simulink model "multiRobotWarehouseVFH"  (R2020b)
settings: Solver=VariableStepAuto  StartTime=0.0  StopTime=inf  RelTol=1e-3
values from neighbouring files (symbols this model uses):
  chargingStations = [90,15;90,25;90,37;90,50;90,60]    [example.m]    (also in warehouseInitial.mat = [90  15; 90  25; 90  37; 90  50; 90  60])
  loadingStations = [70,55;58,21;65,5;47,5;40,30]    [example.m]    (also in warehouseInitial.mat = [70  55; 58  21; 65  5; 47  5; 40  30])
  logicalObsMap = logical(getOccupancy(opmap) + mapMatrix)    [createOBS.m]    (also in example.m = createOBS(logicalMap, obstacle, inflation_num); warehouseInitial.mat = [1 1 1 1 1 1 1 1 1 1 1 1 ... (10000 elements, 100x100)])
  numRobots = size(robotPoses, 2)    [VisualizeWarehouseRobots.m]    (also in example.m = size(chargingStations,1); showresult.m; warehouseInitial.mat = 5)
  obstacle = [35,30]    [example.m]    (also in warehouseInitial.mat = [35 30])
  packages = [1,3,4,5,2]    [example.m]    (also in warehouseInitial.mat = [1 3 4 5 2])
  unloadingStations = [20,58;20,72;10,78;30,78;20,92]    [example.m]    (also in warehouseInitial.mat = [20  58; 20  72; 10  78; 30  78; 20  92])
undefined symbols (not defined in the file or in its folder): RobotState
libraries: robotmobilelib x5
settings Model: Creator=fan  LastModifiedBy=fan

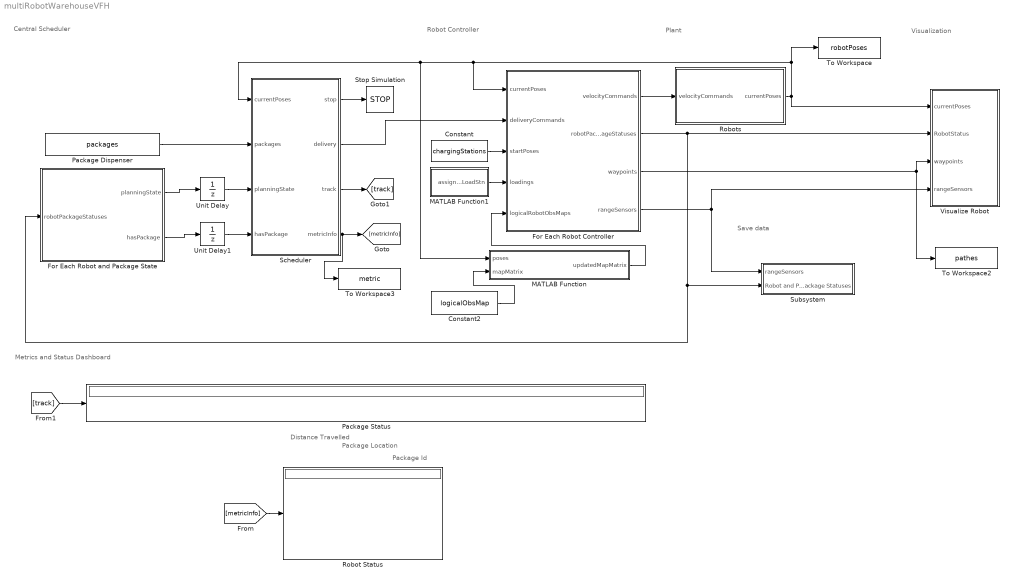
== system multiRobotWarehouseVFH ==
  note: Plant
  note: Package
      | Location
  note: Robot Controller
  note: Metrics and Status Dashboard
  note: Save data
  note: Visualization
  note: Package Id
  note: Distance
      | Travelled
  note: Central Scheduler
  Constant : Constant  Value=chargingStations
  Constant2 : Constant  Value=logicalObsMap
  For Each Robot Controller : Subsystem  TreatAsAtomicUnit=on
  For Each Robot and Package State : Subsystem  TreatAsAtomicUnit=on
  MATLAB Function : MATLAB Function  TreatAsAtomicUnit=on
  MATLAB Function1 : MATLAB Function  TreatAsAtomicUnit=on
  Package Dispenser : Constant  Value=packages
  "Package Status " : Display
  Robot Status : Display
  Robots : Subsystem
  Scheduler : Stateflow chart  Priority=1  TreatAsAtomicUnit=on
  Stop Simulation : Stop
  Subsystem : Subsystem
  To Workspace : ToWorkspace  VariableName=robotPoses  SampleTime=-1
  To Workspace2 : ToWorkspace  VariableName=pathes  SampleTime=-1
  To Workspace3 : ToWorkspace  VariableName=metric  SampleTime=-1
  Unit Delay : UnitDelay  InitialCondition=repmat(RobotState.AtDock, [1, numRobots])  SampleTime=-1  HasFrameUpgradeWarning=on
  Unit Delay1 : UnitDelay  InitialCondition=repmat(0, [1, numRobots])  SampleTime=-1  HasFrameUpgradeWarning=on
  Visualize Robot : Subsystem  mask{MeshSelectionIdx=Ground vehicle, PresetViews=Entire Map, ShowViz=on, ShowPaths=on, MapXMin=0, MapXMax=100, MapYMin=0, MapYMax=100, XLimits=[0 100], YLimits=[0 100], LocalXLimits=[-10 10], LocalYLimits=[-10 10], StartLocations=chargingStations, DockLocations=loadingStations, ShelfLocations=unloadingStations, ObstacleLocation=obstacle, VisualizationSampleRate=10}
      mask prompts: MeshSelectionIdx "Robot mesh"; PresetViews "Preset Views"; ShowViz "Update visualization:"; ShowPaths "Show planned paths:"; MapXMin "Map xmin:"; MapXMax "Map xmax:"; MapYMin "Map ymin:"; MapYMax "Map ymax:"; XLimits "Map x-limits:"; YLimits "Map y-limits:"; LocalXLimits "Local view x-limits"; LocalYLimits "Local view y-limits"; StartLocations "Start locations:"; DockLocations "Dock locations:"; ShelfLocations "Shelf locations:"; ObstacleLocation "Obstacle location:"; VisualizationSampleRate "Sample time:"
      mask init:
      | % Create the list of key locations
      | startLocationMatrix = evalin('base', get_param(gcb, 'StartLocations'));
      | shelfLocationMatrix = evalin('base', get_param(gcb, 'ShelfLocations'));
      | dockLocationMatrix = evalin('base', get_param(gcb, 'DockLocations'));
      | 
      | % Create popup list from matrices
      | dockLocationNameCell = cell(size(dockLocationMatrix,1),1);
      | shelfLocationNameCell = cell(size(shelfLocationMatrix,1),1);
      | startLocationNameCell = cell(size(startLocationMatrix,1),1);
      | for i = 1:size(startLocationMatrix,1)
      |     startLocationNameCell{i} = ['Start Location ' num2str(i)];
      | end
      | for j = 1:size(shelfLocationMatrix,1)
      |     shelfLocationNameCell{j} = ['Shelf Location ' num2str(j)];
      | end
      | for k = 1:size(dockLocationMatrix,1)
      |     dockLocationNameCell{k} = ['Dock Location ' num2str(k)];
      | end
      | 
      | % Update the parameter list
      | m = Simulink.Mask.get(gcb);
      | viewPopupParam = m.getParameter('PresetViews');
      | viewPopupParam.TypeOptions = [...
      |     {'Entire Map'}; ...
      |     dockLocationNameCell; ...
      |     shelfLocationNameCell; ...
      |     startLocationNameCell ... 
      |     ];
      mask TypeOptions MeshSelectionIdx: Ground vehicle | Forklift
      mask TypeOptions PresetViews: Entire Map | Dock Location 1 | Dock Location 2 | Dock Location 3 | Dock Location 4 | Dock Location 5 | Shelf Location 1 | Shelf Location 2 | Shelf Location 3 | Shelf Location 4 | Shelf Location 5 | Start Location 1 | Start Location 2 | Start Location 3 | Start Location 4 | Start Location 5
      mask Callback PresetViews:
      | % Get key numeric data
      | startLocationMatrix = evalin('base', get_param(gcb, 'StartLocations'));
      | dockLocationMatrix = evalin('base', get_param(gcb, 'DockLocations'));
      | shelfLocationMatrix = evalin('base', get_param(gcb, 'ShelfLocations'));
      | mapXLim = evalin('base', get_param(gcb, 'XLimits'));
      | mapYLim = evalin('base', get_param(gcb, 'YLimits'));
      | viewXLim = evalin('base', get_param(gcb, 'LocalXLimits'));
      | viewYLim = evalin('base', get_param(gcb, 'LocalYLimits'));
      | 
      | % Get selected value
      | viewSelection = get_param(gcb, 'PresetViews');
      | 
      | % Take action based on view
      | if strcmp(viewSelection, 'Custom')
      |     % Do nothing
      | else
      |     if strcmp(viewSelection(1:5), 'Start')
      |         % Start location
      |         startIndex = str2double(viewSelection(16:end));
      |         localPts = startLocationMatrix(startIndex, :);
      |         viewLimits = [localPts(1)+viewXLim(1) localPts(1)+viewXLim(2) ...
      |             localPts(2)+viewYLim(1) localPts(2)+viewYLim(2)];
      | 
      |     elseif strcmp(viewSelection(1:5), 'Dock ')
      |         % Dock (Loading) location
      |         dockIndex = str2double(viewSelection(15:end));
      |         localPts = dockLocationMatrix(dockIndex, :);
      |         viewLimits = [localPts(1)+viewXLim(1) localPts(1)+viewXLim(2) ...
      |             localPts(2)+viewYLim(1) localPts(2)+viewYLim(2)];
      | 
      |     elseif strcmp(viewSelection(1:5), 'Shelf')
      |         % Shelf (Unloading) location
      |         shelfIndex = str2double(viewSelection(16:end));
      |         localPts = shelfLocationMatrix(shelfIndex, :);
      |         viewLimits = [localPts(1)+viewXLim(1) localPts(1)+viewXLim(2) ...
      |             localPts(2)+viewYLim(1) localPts(2)+viewYLim(2)];
      | 
      |     else
      |         % Show the whole map
      |         viewLimits = [mapXLim(1) mapXLim(2) mapYLim(1) mapYLim(2)];
      |     end
      | 
      |     % Set the map parameters
      |     set_param(gcb, 'MapXMin', num2str(viewLimits(1)));
      |     set_param(gcb, 'MapXMax', num2str(viewLimits(2)));
      |     set_param(gcb, 'MapYMin', num2str(viewLimits(3)));
      |     set_param(gcb, 'MapYMax', num2str(viewLimits(4)));
      | end
      mask Callback MapXMin:
      | currentMax = str2num(get_param(gcb, 'MapXMax'));
      | newMin = str2num(get_param(gcb, 'MapXMin'));
      | if newMin > currentMax
      |     set_param(gcb, 'MapXMax', num2str(newMin+1));
      | end
      mask Callback MapXMax:
      | currentMin = str2num(get_param(gcb, 'MapXMin'));
      | newMax = str2num(get_param(gcb, 'MapXMax'));
      | if newMax < currentMin
      |     set_param(gcb, 'MapXMin', num2str(newMax-1));
      | end
      mask Callback MapYMin:
      | currentMax = str2num(get_param(gcb, 'MapYMax'));
      | newMin = str2num(get_param(gcb, 'MapYMin'));
      | if newMin > currentMax
      |     set_param(gcb, 'MapYMax', num2str(newMin+1));
      | end
      mask Callback MapYMax:
      | currentMin = str2num(get_param(gcb, 'MapYMin'));
      | newMax = str2num(get_param(gcb, 'MapYMax'));
      | if newMax < currentMin
      |     set_param(gcb, 'MapYMin', num2str(newMax-1));
      | end
      mask DialogControl DescGroupVar Prompt: Visualization example helper
      mask DialogControl DescTextVar Prompt: This subsystem plots the robots and environement and allows users to change the views.
      mask DialogControl ViewLimits Prompt: View limits
      mask DialogControl ViewConfigurationGroup Prompt: View configuration:
      mask DialogControl ViewParamSourcesGroup Prompt: View parameter sources
      mask Display: disp('Visualization Helper')
  wires:
  For Each Robot Controller/4(rangeSensors) -> Subsystem/1(rangeSensors), Visualize Robot/4(rangeSensors)
  Constant2/1 -> MATLAB Function/2(mapMatrix)
  For Each Robot Controller/1(velocityCommands) -> Robots/1(velocityCommands)
  Scheduler/2(delivery) -> For Each Robot Controller/2(deliveryCommands)
  MATLAB Function1/1(assignedLoadStn) -> For Each Robot Controller/4(loadings)
  Unit Delay/1 -> Scheduler/3(planningState)
  For Each Robot and Package State/2(hasPackage) -> Unit Delay1/1
  Unit Delay1/1 -> Scheduler/4(hasPackage)
  [track] -> "Package Status "/1
  Package Dispenser/1 -> Scheduler/2(packages)
  For Each Robot and Package State/1(planningState) -> Unit Delay/1
  Scheduler/1(stop) -> Stop Simulation/1
  For Each Robot Controller/2(robotPackageStatuses) -> Visualize Robot/2(RobotStatus), For Each Robot and Package State/1(robotPackageStatuses), Subsystem/2(Robot and Package Statuses)
  Scheduler/4(metricInfo) -> To Workspace3/1, [metricInfo]
  Constant/1 -> For Each Robot Controller/3(startPoses)
  For Each Robot Controller/3(waypoints) -> To Workspace2/1, Visualize Robot/3(waypoints)
  MATLAB Function/1(updatedMapMatrix) -> For Each Robot Controller/5(logicalRobotObsMaps)
  Robots/1(currentPoses) -> Visualize Robot/1(currentPoses), To Workspace/1, MATLAB Function/1(poses), Scheduler/1(currentPoses), For Each Robot Controller/1(currentPoses)
  [metricInfo] -> Robot Status/1
  Scheduler/3(track) -> [track]

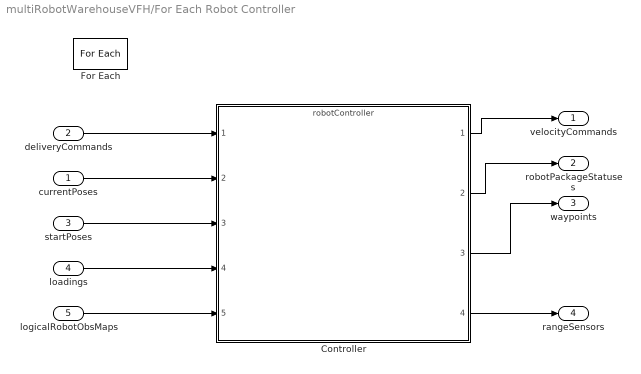
== system multiRobotWarehouseVFH/For Each Robot Controller ==
  currentPoses : Inport  Partition=on  PartitionDimension=2  PartitionWidth=1  PartitionOffset=0
  deliveryCommands : Inport  Port=2  Partition=on  PartitionDimension=1  PartitionWidth=1  PartitionOffset=0
  startPoses : Inport  Port=3  Partition=on  PartitionDimension=1  PartitionWidth=1  PartitionOffset=0
  loadings : Inport  Port=4  Partition=on  PartitionDimension=1  PartitionWidth=1  PartitionOffset=0
  logicalRobotObsMaps : Inport  Port=5  OutDataTypeStr=boolean
  Controller : ModelReference  ModelNameDialog=robotController.slx  ModelReferenceVersion=1.160
  For Each : ForEach  DisableCoverage=on
  velocityCommands : Outport  ConcatenationDimension=2
  robotPackageStatuses : Outport  Port=2  ConcatenationDimension=1
  waypoints : Outport  Port=3  ConcatenationDimension=3
  rangeSensors : Outport  Port=4  ConcatenationDimension=1
  wires:
  deliveryCommands/1 -> Controller/1
  currentPoses/1 -> Controller/2
  startPoses/1 -> Controller/3
  Controller/1 -> velocityCommands/1
  Controller/2 -> robotPackageStatuses/1
  Controller/3 -> waypoints/1
  loadings/1 -> Controller/4
  logicalRobotObsMaps/1 -> Controller/5
  Controller/4 -> rangeSensors/1

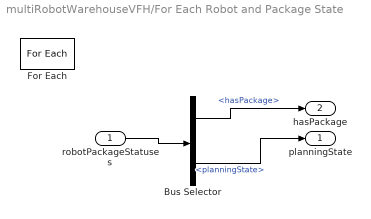
== system multiRobotWarehouseVFH/For Each Robot and Package State ==
  robotPackageStatuses : Inport  Partition=on  PartitionDimension=1  PartitionWidth=1  PartitionOffset=0
  Bus Selector : BusSelector  OutputSignals=hasPackage,planningState
  For Each : ForEach  DisableCoverage=on
  planningState : Outport  ConcatenationDimension=1
  hasPackage : Outport  Port=2  ConcatenationDimension=1
  wires:
  robotPackageStatuses/1 -> Bus Selector/1
  Bus Selector/1 -> hasPackage/1  "<hasPackage>"
  Bus Selector/2 -> planningState/1  "<planningState>"

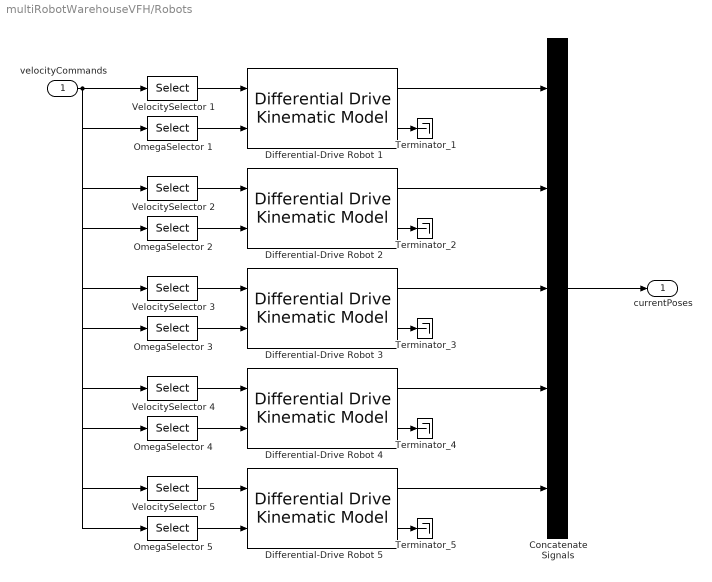
== system multiRobotWarehouseVFH/Robots ==
  velocityCommands : Inport
  Concatenate Signals : Concatenate  NumInputs=5  Mode=Multidimensional array  ConcatenateDimension=2
  Differential-Drive Robot 1 : robotmobilelib/Differential Drive Kinematic Model  VehicleInputs=Vehicle Speed & Heading Angular Velocity  WheelRadius=0.1  WheelSpeedRange=[-inf inf]  TrackWidth=0.2  InitialState=[chargingStations(1, :), 0]'  SimulateUsing=Interpreted execution
      settings: SourceProductName=Robotics System Toolbox
  Differential-Drive Robot 2 : robotmobilelib/Differential Drive Kinematic Model  VehicleInputs=Vehicle Speed & Heading Angular Velocity  WheelRadius=0.1  WheelSpeedRange=[-inf inf]  TrackWidth=0.2  InitialState=[chargingStations(2, :), 0]'  SimulateUsing=Interpreted execution
      settings: SourceProductName=Robotics System Toolbox
  Differential-Drive Robot 3 : robotmobilelib/Differential Drive Kinematic Model  VehicleInputs=Vehicle Speed & Heading Angular Velocity  WheelRadius=0.1  WheelSpeedRange=[-inf inf]  TrackWidth=0.2  InitialState=[chargingStations(3, :), 0]'  SimulateUsing=Interpreted execution
      settings: SourceProductName=Robotics System Toolbox
  Differential-Drive Robot 4 : robotmobilelib/Differential Drive Kinematic Model  VehicleInputs=Vehicle Speed & Heading Angular Velocity  WheelRadius=0.1  WheelSpeedRange=[-inf inf]  TrackWidth=0.2  InitialState=[chargingStations(4, :), 0]'  SimulateUsing=Interpreted execution
      settings: SourceProductName=Robotics System Toolbox
  Differential-Drive Robot 5 : robotmobilelib/Differential Drive Kinematic Model  VehicleInputs=Vehicle Speed & Heading Angular Velocity  WheelRadius=0.1  WheelSpeedRange=[-inf inf]  TrackWidth=0.2  InitialState=[chargingStations(5, :), 0]'  SimulateUsing=Interpreted execution
      settings: SourceProductName=Robotics System Toolbox
  OmegaSelector 1 : Selector  NumberOfDimensions=2  InputPortWidth=3  IndexOptions=Index vector (dialog),Index vector (dialog)  Indices=2,1  OutputSizes=1
  OmegaSelector 2 : Selector  NumberOfDimensions=2  InputPortWidth=3  IndexOptions=Index vector (dialog),Index vector (dialog)  Indices=2,2  OutputSizes=1
  OmegaSelector 3 : Selector  NumberOfDimensions=2  InputPortWidth=3  IndexOptions=Index vector (dialog),Index vector (dialog)  Indices=2,3  OutputSizes=1
  OmegaSelector 4 : Selector  NumberOfDimensions=2  InputPortWidth=3  IndexOptions=Index vector (dialog),Index vector (dialog)  Indices=2,4  OutputSizes=1
  OmegaSelector 5 : Selector  NumberOfDimensions=2  InputPortWidth=3  IndexOptions=Index vector (dialog),Index vector (dialog)  Indices=2,5  OutputSizes=1
  Terminator_{1..5} (5 alike) : Terminator
  VelocitySelector 1 : Selector  NumberOfDimensions=2  InputPortWidth=3  IndexOptions=Index vector (dialog),Index vector (dialog)  Indices=1,1  OutputSizes=1
  VelocitySelector 2 : Selector  NumberOfDimensions=2  InputPortWidth=3  IndexOptions=Index vector (dialog),Index vector (dialog)  Indices=1,2  OutputSizes=1
  VelocitySelector 3 : Selector  NumberOfDimensions=2  InputPortWidth=3  IndexOptions=Index vector (dialog),Index vector (dialog)  Indices=1,3  OutputSizes=1
  VelocitySelector 4 : Selector  NumberOfDimensions=2  InputPortWidth=3  IndexOptions=Index vector (dialog),Index vector (dialog)  Indices=1,4  OutputSizes=1
  VelocitySelector 5 : Selector  NumberOfDimensions=2  InputPortWidth=3  IndexOptions=Index vector (dialog),Index vector (dialog)  Indices=1,5  OutputSizes=1
  currentPoses : Outport
  wires:
  Concatenate Signals/1 -> currentPoses/1
  velocityCommands/1 -> VelocitySelector 1/1, OmegaSelector 1/1, VelocitySelector 2/1, OmegaSelector 2/1, VelocitySelector 3/1, OmegaSelector 3/1, VelocitySelector 4/1, OmegaSelector 4/1, VelocitySelector 5/1, OmegaSelector 5/1
  VelocitySelector 1/1 -> Differential-Drive Robot 1/1
  OmegaSelector 1/1 -> Differential-Drive Robot 1/2
  Differential-Drive Robot 1/1 -> Concatenate Signals/1
  VelocitySelector 2/1 -> Differential-Drive Robot 2/1
  OmegaSelector 2/1 -> Differential-Drive Robot 2/2
  Differential-Drive Robot 2/1 -> Concatenate Signals/2
  VelocitySelector 3/1 -> Differential-Drive Robot 3/1
  OmegaSelector 3/1 -> Differential-Drive Robot 3/2
  Differential-Drive Robot 3/1 -> Concatenate Signals/3
  VelocitySelector 4/1 -> Differential-Drive Robot 4/1
  OmegaSelector 4/1 -> Differential-Drive Robot 4/2
  Differential-Drive Robot 4/1 -> Concatenate Signals/4
  VelocitySelector 5/1 -> Differential-Drive Robot 5/1
  OmegaSelector 5/1 -> Differential-Drive Robot 5/2
  Differential-Drive Robot 5/1 -> Concatenate Signals/5
  Differential-Drive Robot 1/2 -> Terminator_1/1
  Differential-Drive Robot 2/2 -> Terminator_2/1
  Differential-Drive Robot 3/2 -> Terminator_3/1
  Differential-Drive Robot 4/2 -> Terminator_4/1
  Differential-Drive Robot 5/2 -> Terminator_5/1

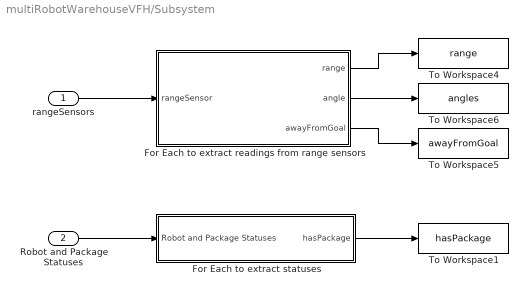
== system multiRobotWarehouseVFH/Subsystem ==
  rangeSensors : Inport
  Robot and Package Statuses : Inport  Port=2
  For Each to extract readings from range sensors : Subsystem  TreatAsAtomicUnit=on
  For Each to extract statuses : Subsystem  TreatAsAtomicUnit=on
  To Workspace1 : ToWorkspace  VariableName=hasPackage  SampleTime=-1
  To Workspace4 : ToWorkspace  VariableName=range  SampleTime=-1
  To Workspace5 : ToWorkspace  VariableName=awayFromGoal  SampleTime=-1
  To Workspace6 : ToWorkspace  VariableName=angles  SampleTime=-1
  wires:
  For Each to extract readings from range sensors/2(angle) -> To Workspace6/1
  For Each to extract readings from range sensors/3(awayFromGoal) -> To Workspace5/1
  For Each to extract readings from range sensors/1(range) -> To Workspace4/1
  rangeSensors/1 -> For Each to extract readings from range sensors/1(rangeSensor)
  For Each to extract statuses/1(hasPackage) -> To Workspace1/1
  Robot and Package Statuses/1 -> For Each to extract statuses/1(Robot and Package Statuses)

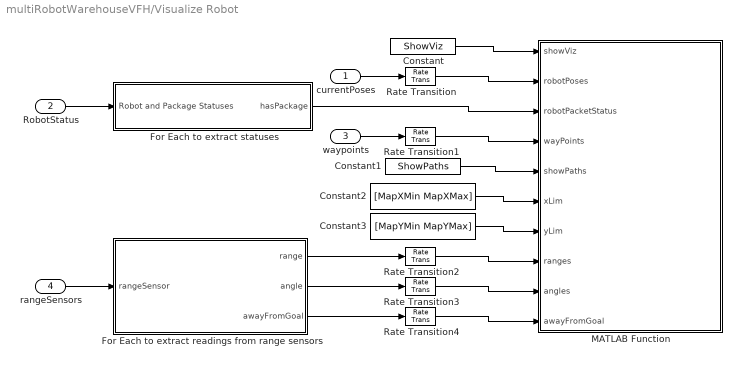
== system multiRobotWarehouseVFH/Visualize Robot ==
  currentPoses : Inport
  RobotStatus : Inport  Port=2
  waypoints : Inport  Port=3
  rangeSensors : Inport  Port=4
  Constant : Constant  Value=ShowViz
  Constant1 : Constant  Value=ShowPaths
  Constant2 : Constant  Value=[MapXMin MapXMax]
  Constant3 : Constant  Value=[MapYMin MapYMax]
  For Each to extract readings from range sensors : Subsystem  TreatAsAtomicUnit=on
  For Each to extract statuses : Subsystem  TreatAsAtomicUnit=on
  MATLAB Function : MATLAB Function  TreatAsAtomicUnit=on
  Rate Transition{,1..4} (5 alike) : RateTransition
  wires:
  waypoints/1 -> Rate Transition1/1
  currentPoses/1 -> Rate Transition/1
  Rate Transition/1 -> MATLAB Function/2(robotPoses)
  Rate Transition1/1 -> MATLAB Function/4(wayPoints)
  Constant/1 -> MATLAB Function/1(showViz)
  Constant1/1 -> MATLAB Function/5(showPaths)
  Constant2/1 -> MATLAB Function/6(xLim)
  Constant3/1 -> MATLAB Function/7(yLim)
  RobotStatus/1 -> For Each to extract statuses/1(Robot and Package Statuses)
  For Each to extract statuses/1(hasPackage) -> MATLAB Function/3(robotPacketStatus)
  For Each to extract readings from range sensors/1(range) -> Rate Transition2/1
  Rate Transition2/1 -> MATLAB Function/8(ranges)
  Rate Transition3/1 -> MATLAB Function/9(angles)
  For Each to extract readings from range sensors/2(angle) -> Rate Transition3/1
  Rate Transition4/1 -> MATLAB Function/10(awayFromGoal)
  For Each to extract readings from range sensors/3(awayFromGoal) -> Rate Transition4/1
  rangeSensors/1 -> For Each to extract readings from range sensors/1(rangeSensor)

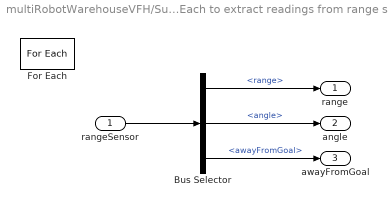
== system multiRobotWarehouseVFH/Subsystem/For Each to extract readings from range sensors ==
  rangeSensor : Inport  Partition=on  PartitionDimension=1  PartitionWidth=1  PartitionOffset=0
  Bus Selector : BusSelector  OutputSignals=range,angle,awayFromGoal
  For Each : ForEach  DisableCoverage=on
  range : Outport  ConcatenationDimension=2
  angle : Outport  Port=2  ConcatenationDimension=2
  awayFromGoal : Outport  Port=3  OutDataTypeStr=boolean  ConcatenationDimension=1
  wires:
  rangeSensor/1 -> Bus Selector/1
  Bus Selector/1 -> range/1  "<range>"
  Bus Selector/2 -> angle/1  "<angle>"
  Bus Selector/3 -> awayFromGoal/1  "<awayFromGoal>"

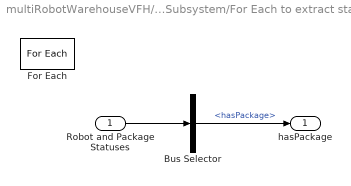
== system multiRobotWarehouseVFH/Subsystem/For Each to extract statuses ==
  Robot and Package Statuses : Inport  Partition=on  PartitionDimension=1  PartitionWidth=1  PartitionOffset=0
  Bus Selector : BusSelector  OutputSignals=hasPackage
  For Each : ForEach  DisableCoverage=on
  hasPackage : Outport  ConcatenationDimension=1
  wires:
  Robot and Package Statuses/1 -> Bus Selector/1
  Bus Selector/1 -> hasPackage/1  "<hasPackage>"

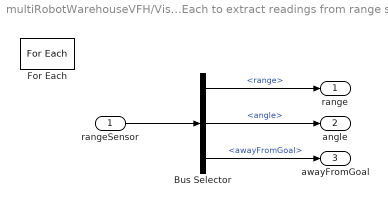
== system multiRobotWarehouseVFH/Visualize Robot/For Each to extract readings from range sensors ==
  rangeSensor : Inport  Partition=on  PartitionDimension=1  PartitionWidth=1  PartitionOffset=0
  Bus Selector : BusSelector  OutputSignals=range,angle,awayFromGoal
  For Each : ForEach  DisableCoverage=on
  range : Outport  ConcatenationDimension=2
  angle : Outport  Port=2  ConcatenationDimension=2
  awayFromGoal : Outport  Port=3  OutDataTypeStr=boolean  ConcatenationDimension=1
  wires:
  rangeSensor/1 -> Bus Selector/1
  Bus Selector/1 -> range/1  "<range>"
  Bus Selector/2 -> angle/1  "<angle>"
  Bus Selector/3 -> awayFromGoal/1  "<awayFromGoal>"

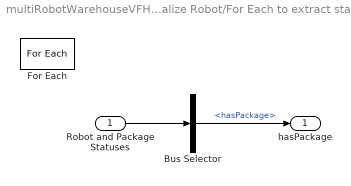
== system multiRobotWarehouseVFH/Visualize Robot/For Each to extract statuses ==
  Robot and Package Statuses : Inport  Partition=on  PartitionDimension=1  PartitionWidth=1  PartitionOffset=0
  Bus Selector : BusSelector  OutputSignals=hasPackage
  For Each : ForEach  DisableCoverage=on
  hasPackage : Outport  ConcatenationDimension=1
  wires:
  Robot and Package Statuses/1 -> Bus Selector/1
  Bus Selector/1 -> hasPackage/1  "<hasPackage>"

== matlab function multiRobotWarehouseVFH/MATLAB Function ==
  settings: updateMethod=DISCRETE
  data: poses input; mapMatrix input; updatedMapMatrix output boolean
function updatedMapMatrix = updateMap(poses,mapMatrix)

posesMap = zeros(size(mapMatrix));
% num_robot = size(poses,1);
poses_grid = world2grid(binaryOccupancyMap(mapMatrix), poses(1:2,:)');
idx = sub2ind(size(mapMatrix),poses_grid(:,1),poses_grid(:,2));
posesMap(idx) = true;
updatedMapMatrix = logical(posesMap + mapMatrix);


end

== matlab function multiRobotWarehouseVFH/Visualize Robot/MATLAB Function ==
  settings: updateMethod=DISCRETE  sampleTime=VisualizationSampleRate
  data: showViz input; robotPoses input; robotPacketStatus input; wayPoints input; ShelfLocations parameter; DockLocations parameter; showPaths input; xLim input; yLim input; MeshSelectionIdx parameter; ranges input; angles input; awayFromGoal input; StartLocations parameter; ObstacleLocation parameter; logicalObsMap parameter
function simulationVisualization(showViz, robotPoses, robotPacketStatus, wayPoints, ShelfLocations, DockLocations, showPaths, xLim, yLim, MeshSelectionIdx, ranges, angles, awayFromGoal, StartLocations, ObstacleLocation, logicalObsMap)
%#codegen

%% Setup

coder.extrinsic('VisualizeWarehouseRobots');
persistent f

if isempty(f) && showViz
    f = figure('units','normalized','outerposition',[0 0 0.75 0.75]);
%     ax = axes('Parent', f);
    title('Mobile Robot Motion');
    set(f, 'Visible', 'on');
end

% Robot mesh options are cells of the unloaded and loaded robot mesh and
% the translation between the visualized origin and the desired origin
meshOptions = {...
    {'groundvehicle.stl', [.314 0 .155], 'groundvehiclewithload.stl', [.312 0 .156]}, ...
    {'forklift.stl', [.3569 0 .297], 'forkliftwithload.stl', [.3813 0 .2893]}, ...
    };
    

if showViz
    VisualizeWarehouseRobots(robotPoses, robotPacketStatus, wayPoints, logicalObsMap, StartLocations, ShelfLocations, DockLocations, ObstacleLocation, showPaths, xLim, yLim, meshOptions{MeshSelectionIdx}, ranges, angles, awayFromGoal);
end

end

== stateflow chart multiRobotWarehouseVFH/Scheduler ==
  settings: sampleTime=0.1
  state Assign
    entry:
    stop = 0;
    Assign -> (junction 258) [order 1] : [currentPackage <= length(packages)]{robot = 1;}
    (junction 258) -> (junction 257) [order 1] : [robot <= numRobots]
    (junction 257) -> (junction 391) [order 1] : [planningState(robot) == RobotState.AtLoadingStn && ...
        | ~hasPackage(robot)&&...
        | currentPackage <= length(packages)]
        | {
        | delivery(robot).package= packages(robot);
        | delivery(robot).packageId = currentPackage;
        | currentPackage = currentPackage + 1;
        | delivery(robot).givenPackage = 1;
        | }
    (junction 258) -> (junction 398) [order 2] : {packageTrack;
        | robotTrack;}
    (junction 393) -> (junction 258)
    (junction 257) -> (junction 259) [order 2] : {delivery(robot).givenPackage = 0;}
    (junction 391) -> (junction 332)
    (junction 259) -> (junction 393) : {robot = robot + 1;}
    (junction 332) -> (junction 259)
  state LastPackage
    LastPackage -> (junction 344) [order 1] : {robot = 1;}
    (junction 344) -> (junction 343) [order 1] : [robot <= numRobots]
    (junction 344) -> (junction 426) [order 2] : {packageTrack;
        | robotTrack;}
    (junction 346) -> (junction 344)
    (junction 343) -> (junction 345) : {delivery(robot).givenPackage = 0;
        | }
    (junction 345) -> (junction 346) : {robot = robot + 1;}
  state Stop
    stop = 1;
  (default) -> Assign
  Assign -> LastPackage [order 1] : [currentPackage > length(packages)]
      | {packageTrack;
      | robotTrack;}
  Stop -> (junction 351)
  LastPackage -> Stop [order 1] : [all(planningState==RobotState.AtDock)]{
      | robotTrack;
      | packageTrack;}
  data: currentPoses input; packages input; planningState input; robot local =1; stop output; currentPackage local =1; hasPackage input; numRobots local =size(chargingStations, 1); delivery output Bus: RobotDeliverCommand size=numRobots; track output Enum: PackageState size=[1, length(packets)] =repmat(PackageState.Unassigned, 1, length(packages)); prevPose local =chargingStations'; metricInfo output =zeros(numRobots, 3); distance local =zeros(numRobots, 1)
  function packageTrack:
    | function packageTrack
    | numPackets = length(packages);
    | for r = 1 : numRobots
    |     packageId = delivery(r).packageId;
    |     if(packageId > 0 && track(packageId) ~= PackageState.Delivered)
    |         track(packageId) = PackageState.InProgress;
    |     end
    |     if(packageId > 0)
    |         if(~hasPackage(r) && planningState(r) == RobotState.AtUnloadingStn)
    |             track(packageId) = PackageState.Delivered;
    |         end
    |     end
    | end
  function robotTrack:
    | function robotTrack
    | % calculate distance
    | displacement = (prevPose - currentPoses(1:2, :));
    | d = sqrt(diag(displacement' * displacement));
    | distance = distance + d;
    | prevPose = currentPoses(1:2, :);
    | d = distance;
    | metricInfo(:, 1) = distance(:);
    | 
    | robotPackages = zeros(1, numRobots);
    | robotPackageId = zeros(1, numRobots);
    | packetIds = zeros(1, numRobots);
    | for r = 1:numRobots
    |     robotPackages(r) = delivery(r).package;
    |     robotPackageId(r) = delivery(r).packageId;
    | end
    | metricInfo(:, 2) = robotPackages(:);
    | metricInfo(:, 3) = robotPackageId(:);
    | end

== matlab function multiRobotWarehouseVFH/MATLAB Function1 ==
  data: assignedLoadStn output; loadingStations parameter; packages parameter
function assignedLoadStn = assignLoadStn(loadingStations, packages)
assignedLoadStn = zeros(size(loadingStations));
for i=1:size(packages,2)
    assignedLoadStn(i,:) = loadingStations(packages(i),:);
end

end
